simulink model "xpc_dlt_adept_sa_1"  (R2013b)
settings: Solver=ode4  StartTime=0.0  StopTime=4  FixedStep=0.001  RelTol=1e-3
libraries: xpcnilib x6, xpclib x4, simulink x3
(part 1 of 2)
settings Model: BufferReuse=off  Creator=lucius  LastModifiedBy=lucius
settings OptimizationCC: BlockReduction=off  OptimizeBlockIOStorage=off  BufferReuse=off  ExpressionFolding=off  LocalBlockOutputs=off
settings HardwareCC: ProdIntDivRoundTo=Zero  ProdEndianess=LittleEndian  ProdHWDeviceType=Generic->32-bit x86 compatible
settings RTWCC: SystemTargetFile=xpctarget.tlc  TemplateMakefile=xpc_default_tmf  Description=xPC Target  ProcessScript=xpctarget_make_rtw_hook  RTWCompilerOptimization=On
settings xpcTargetCC: TargetFcnLib=ansi_tfl_table_tmw.mat  CodeReplacementLibrary=XPC_BLAS  ParMdlRefBuildCompliant=on  ConcurrentExecutionCompliant=on  CombineSignalStateStructs=off  MATLABClassNameForMDSCustomization=xpcAperiodicCustomization  GRTInterface=on  GenerateAllocFcn=off  xPCTaskExecutionProfile=off  xPCRL32EventNumber=5000  xPCLoadParamSetFile=off  xPCConcurrentTasks=off  xPCEnableSFAnimation=off

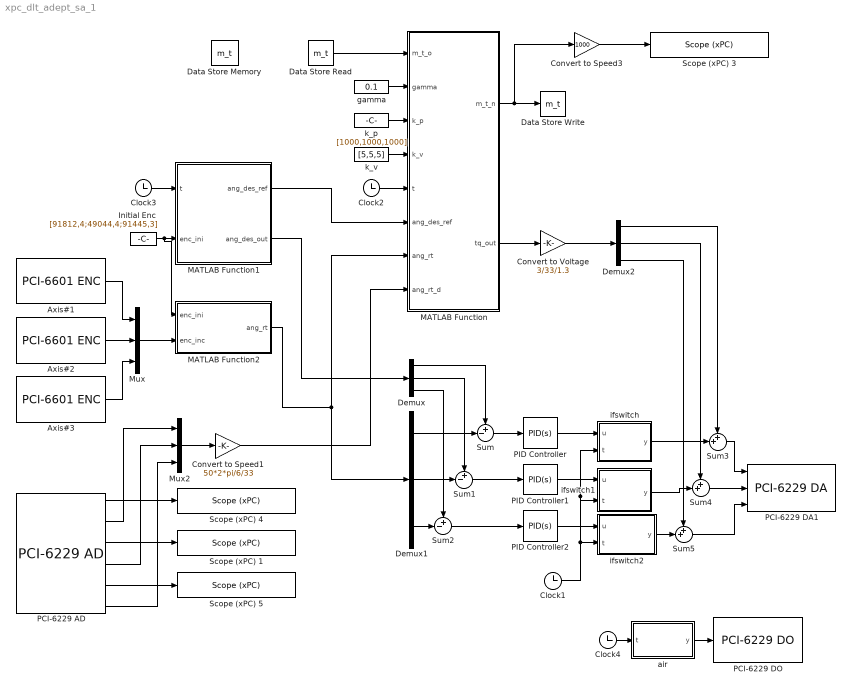
== system xpc_dlt_adept_sa_1 ==
  Axis#1 : xpcnilib/Incremental Encoder/PCI-6601 ENC  channel=1  countMode=Quadrature Mode X4  initCount=0  reload=off  indexPhase=A low B low  filter=None  sampleTime=0.001  slot=-1
  Axis#2 : xpcnilib/Incremental Encoder/PCI-6601 ENC  channel=2  countMode=Quadrature Mode X4  initCount=0  reload=off  indexPhase=A low B low  filter=None  sampleTime=0.001  slot=-1
  Axis#3 : xpcnilib/Incremental Encoder/PCI-6601 ENC  channel=3  countMode=Quadrature Mode X4  initCount=0  reload=off  indexPhase=A low B low  filter=None  sampleTime=0.001  slot=-1
  Clock{1..4} (4 alike) : Clock
  Convert to Speed1 : Gain  Gain=50*2*pi/6/33
  Convert to Speed3 : Gain  Gain=1000
  Convert to Voltage : Gain  Gain=3/33/1.3
  Data Store Memory : DataStoreMemory  DataStoreName=m_t  ReadBeforeWriteMsg=warning  WriteAfterWriteMsg=warning  WriteAfterReadMsg=warning
  Data Store Read : DataStoreRead  DataStoreName=m_t
  Data Store Write : DataStoreWrite  DataStoreName=m_t
  Demux : Demux  Outputs=3
  Demux1 : Demux  Outputs=3
  Demux2 : Demux  Outputs=3
  Initial Enc : Constant  Value=[91812,4;49044,4;91445,3]
  MATLAB Function : MATLAB Function  TreatAsAtomicUnit=on
  MATLAB Function1 : MATLAB Function  TreatAsAtomicUnit=on
  MATLAB Function2 : MATLAB Function  TreatAsAtomicUnit=on
  Mux : Mux  Inputs=3
  Mux2 : Mux  Inputs=3
  PCI-6229 AD : xpcnilib/A//D/M Series/PCI-6229 AD  channel=[1,2,3,4,17,18]  range=[10]  coupling=[0]  scantime=5e-6  sampletime=0.001  slot=-1
  PCI-6229 DA1 : xpcnilib/D//A/M Series/PCI-6229 DA  channel=[1,2,3]  reset=[1,1,1]  initValue=[0,0,0]  sampletime=-1  slot=-1
  PCI-6229 DO : xpcnilib/Digital Output/M Series/PCI-6229 DO  channel=[1]  reset=[1]  initValue=[0]  sampletime=0.001  slot=-1
  PID Controller : simulink/Continuous/PID Controller  Controller=PID  TimeDomain=Continuous-time  SampleTime=1  IntegratorMethod=Forward Euler  FilterMethod=Forward Euler  Form=Parallel  P=50  I=60  D=2  N=100  InitialConditionSource=internal  InitialConditionForIntegrator=0  InitialConditionForFilter=0  ExternalReset=none  LimitOutput=off  UpperSaturationLimit=inf  LowerSaturationLimit=-inf  LinearizeAsGain=on  AntiWindupMode=none  Kb=1  TrackingMode=off  Kt=1  PParamMin=[]  PParamMax=[]  IParamMin=[]  IParamMax=[]  DParamMin=[]  DParamMax=[]  NParamMin=[]  NParamMax=[]  KbParamMin=[]  KbParamMax=[]  KtParamMin=[]  KtParamMax=[]  POutMin=[]  POutMax=[]  IOutMin=[]  IOutMax=[]  DOutMin=[]  DOutMax=[]  NOutMin=[]  NOutMax=[]  KbOutMin=[]  KbOutMax=[]  KtOutMin=[]  KtOutMax=[]  IntegratorOutMin=[]  IntegratorOutMax=[]  FilterOutMin=[]  FilterOutMax=[]  SumOutMin=[]  SumOutMax=[]  SumI1OutMin=[]  SumI1OutMax=[]  SumI2OutMin=[]  SumI2OutMax=[]  SumI3OutMin=[]  SumI3OutMax=[]  SumDOutMin=[]  SumDOutMax=[]  SaturationOutMin=[]  SaturationOutMax=[]  IntegratorContinuousStateAttributes=''  IntegratorStateMustResolveToSignalObject=off  IntegratorRTWStateStorageClass=Auto  FilterContinuousStateAttributes=''  FilterStateMustResolveToSignalObject=off  FilterRTWStateStorageClass=Auto
  PID Controller1 : simulink/Continuous/PID Controller  Controller=PID  TimeDomain=Continuous-time  SampleTime=1  IntegratorMethod=Forward Euler  FilterMethod=Forward Euler  Form=Parallel  P=50  I=60  D=2  N=100  InitialConditionSource=internal  InitialConditionForIntegrator=0  InitialConditionForFilter=0  ExternalReset=none  LimitOutput=off  UpperSaturationLimit=inf  LowerSaturationLimit=-inf  LinearizeAsGain=on  AntiWindupMode=none  Kb=1  TrackingMode=off  Kt=1  PParamMin=[]  PParamMax=[]  IParamMin=[]  IParamMax=[]  DParamMin=[]  DParamMax=[]  NParamMin=[]  NParamMax=[]  KbParamMin=[]  KbParamMax=[]  KtParamMin=[]  KtParamMax=[]  POutMin=[]  POutMax=[]  IOutMin=[]  IOutMax=[]  DOutMin=[]  DOutMax=[]  NOutMin=[]  NOutMax=[]  KbOutMin=[]  KbOutMax=[]  KtOutMin=[]  KtOutMax=[]  IntegratorOutMin=[]  IntegratorOutMax=[]  FilterOutMin=[]  FilterOutMax=[]  SumOutMin=[]  SumOutMax=[]  SumI1OutMin=[]  SumI1OutMax=[]  SumI2OutMin=[]  SumI2OutMax=[]  SumI3OutMin=[]  SumI3OutMax=[]  SumDOutMin=[]  SumDOutMax=[]  SaturationOutMin=[]  SaturationOutMax=[]  IntegratorContinuousStateAttributes=''  IntegratorStateMustResolveToSignalObject=off  IntegratorRTWStateStorageClass=Auto  FilterContinuousStateAttributes=''  FilterStateMustResolveToSignalObject=off  FilterRTWStateStorageClass=Auto
  PID Controller2 : simulink/Continuous/PID Controller  Controller=PID  TimeDomain=Continuous-time  SampleTime=1  IntegratorMethod=Forward Euler  FilterMethod=Forward Euler  Form=Parallel  P=50  I=60  D=2  N=100  InitialConditionSource=internal  InitialConditionForIntegrator=0  InitialConditionForFilter=0  ExternalReset=none  LimitOutput=off  UpperSaturationLimit=inf  LowerSaturationLimit=-inf  LinearizeAsGain=on  AntiWindupMode=none  Kb=1  TrackingMode=off  Kt=1  PParamMin=[]  PParamMax=[]  IParamMin=[]  IParamMax=[]  DParamMin=[]  DParamMax=[]  NParamMin=[]  NParamMax=[]  KbParamMin=[]  KbParamMax=[]  KtParamMin=[]  KtParamMax=[]  POutMin=[]  POutMax=[]  IOutMin=[]  IOutMax=[]  DOutMin=[]  DOutMax=[]  NOutMin=[]  NOutMax=[]  KbOutMin=[]  KbOutMax=[]  KtOutMin=[]  KtOutMax=[]  IntegratorOutMin=[]  IntegratorOutMax=[]  FilterOutMin=[]  FilterOutMax=[]  SumOutMin=[]  SumOutMax=[]  SumI1OutMin=[]  SumI1OutMax=[]  SumI2OutMin=[]  SumI2OutMax=[]  SumI3OutMin=[]  SumI3OutMax=[]  SumDOutMin=[]  SumDOutMax=[]  SaturationOutMin=[]  SaturationOutMax=[]  IntegratorContinuousStateAttributes=''  IntegratorStateMustResolveToSignalObject=off  IntegratorRTWStateStorageClass=Auto  FilterContinuousStateAttributes=''  FilterStateMustResolveToSignalObject=off  FilterRTWStateStorageClass=Auto
  Scope (xPC) 1 : xpclib/Misc./Scope (xPC)   scopeno=5  scopetype=File  autostart=on  viewmode=Graphical redraw  formatstr='%15.6f'  grid=on  ylimits=[0,0]  nosamples=4000  noprepostsamples=0  interleave=1  triggermode=FreeRun  triggersignal=1  trigsignalfromport=off  triggerlevel=0.0  triggerslope=Either  triggerscope=1  triggersample=0  filename=a2t23s12.dat  mode=Lazy  writesize=512  autorestart=off  dynamicfilemode=off  maxwritefilesize=512*1024^2
  Scope (xPC) 3 : xpclib/Misc./Scope (xPC)   scopeno=4  scopetype=File  autostart=on  viewmode=Graphical redraw  formatstr='%15.6f'  grid=on  ylimits=[500,1000]  nosamples=4000  noprepostsamples=0  interleave=1  triggermode=FreeRun  triggersignal=1  trigsignalfromport=off  triggerlevel=0.0  triggerslope=Either  triggerscope=1  triggersample=0  filename=p23s12.dat  mode=Lazy  writesize=512  autorestart=off  dynamicfilemode=off  maxwritefilesize=512*1024^2
  Scope (xPC) 4 : xpclib/Misc./Scope (xPC)   scopeno=1  scopetype=File  autostart=on  viewmode=Graphical redraw  formatstr='%15.6f'  grid=on  ylimits=[0,0]  nosamples=4000  noprepostsamples=0  interleave=1  triggermode=FreeRun  triggersignal=1  trigsignalfromport=off  triggerlevel=0.0  triggerslope=Either  triggerscope=1  triggersample=0  filename=a1t23s12.dat  mode=Lazy  writesize=512  autorestart=off  dynamicfilemode=off  maxwritefilesize=512*1024^2
  Scope (xPC) 5 : xpclib/Misc./Scope (xPC)   scopeno=3  scopetype=File  autostart=on  viewmode=Graphical redraw  formatstr='%15.6f'  grid=on  ylimits=[0,0]  nosamples=4000  noprepostsamples=0  interleave=1  triggermode=FreeRun  triggersignal=1  trigsignalfromport=off  triggerlevel=0.0  triggerslope=Either  triggerscope=1  triggersample=0  filename=a3t23s12.dat  mode=Lazy  writesize=512  autorestart=off  dynamicfilemode=off  maxwritefilesize=512*1024^2
  Sum : Sum  Inputs=+-|
  Sum1 : Sum  Inputs=+-|
  Sum2 : Sum  Inputs=+-|
  Sum3 : Sum  Inputs=++|
  Sum4 : Sum  Inputs=++|
  Sum5 : Sum  Inputs=++|
  air : MATLAB Function  TreatAsAtomicUnit=on
  gamma : Constant  Value=0.1
  ifswitch : MATLAB Function  TreatAsAtomicUnit=on
  ifswitch1 : MATLAB Function  TreatAsAtomicUnit=on
  ifswitch2 : MATLAB Function  TreatAsAtomicUnit=on
  k_p : Constant  Value=[1000,1000,1000]
  k_v : Constant  Value=[5,5,5]
  wires:
  Axis#1/1 -> Mux/1
  Axis#2/1 -> Mux/2
  Axis#3/1 -> Mux/3
  Mux/1 -> MATLAB Function2/2(enc_inc)
  Initial Enc/1 -> MATLAB Function2/1(enc_ini), MATLAB Function1/2(enc_ini)
  Clock3/1 -> MATLAB Function1/1(t)
  MATLAB Function1/1(ang_des_ref) -> MATLAB Function/6(ang_des_ref)
  MATLAB Function/2(tq_out) -> Convert to Voltage/1
  Convert to Voltage/1 -> Demux2/1
  k_v/1 -> MATLAB Function/4(k_v)
  k_p/1 -> MATLAB Function/3(k_p)
  Demux/1 -> Sum/1
  Demux/3 -> Sum2/1
  Demux/2 -> Sum1/1
  Sum/1 -> PID Controller/1
  Sum1/1 -> PID Controller1/1
  Sum2/1 -> PID Controller2/1
  Demux1/1 -> Sum/2
  Demux1/2 -> Sum1/2
  Demux1/3 -> Sum2/2
  Demux2/1 -> Sum3/1
  Demux2/3 -> Sum5/1
  Demux2/2 -> Sum4/1
  Sum3/1 -> PCI-6229 DA1/1
  Sum4/1 -> PCI-6229 DA1/2
  Sum5/1 -> PCI-6229 DA1/3
  PID Controller1/1 -> ifswitch1/1(u)
  PID Controller/1 -> ifswitch/1(u)
  PID Controller2/1 -> ifswitch2/1(u)
  Clock1/1 -> ifswitch/2(t), ifswitch1/2(t), ifswitch2/2(t)
  ifswitch/1(y) -> Sum3/2
  ifswitch1/1(y) -> Sum4/2
  ifswitch2/1(y) -> Sum5/2
  MATLAB Function1/2(ang_des_out) -> Demux/1
  MATLAB Function2/1(ang_rt) -> MATLAB Function/7(ang_rt), Demux1/1
  Clock2/1 -> MATLAB Function/5(t)
  air/1(y) -> PCI-6229 DO/1
  Clock4/1 -> air/1(t)
  gamma/1 -> MATLAB Function/2(gamma)
  Mux2/1 -> Convert to Speed1/1
  PCI-6229 AD/3 -> Scope (xPC) 1/1
  PCI-6229 AD/6 -> Mux2/3
  PCI-6229 AD/4 -> Mux2/2
  PCI-6229 AD/2 -> Mux2/1
  Convert to Speed1/1 -> MATLAB Function/8(ang_rt_d)
  MATLAB Function/1(m_t_n) -> Convert to Speed3/1, Data Store Write/1
  Data Store Read/1 -> MATLAB Function/1(m_t_o)
  Convert to Speed3/1 -> Scope (xPC) 3/1
  PCI-6229 AD/1 -> Scope (xPC) 4/1
  PCI-6229 AD/5 -> Scope (xPC) 5/1

== matlab function xpc_dlt_adept_sa_1/ifswitch1 ==
  data: u input; y output; t input
function y = ifswitch(u,t)
T=2;
if t<T
y = u;
else y=0;
end

== matlab function xpc_dlt_adept_sa_1/ifswitch ==
  data: u input; y output; t input
function y = ifswitch(u,t)
T=2;
if t<T
y = u;
else y=0;
end

== matlab function xpc_dlt_adept_sa_1/MATLAB Function2 ==
  data: enc_ini input; ang_rt output; enc_inc input
function ang_rt = inc2jo(enc_ini,enc_inc)
%***********************REFERENCE****************************************
%LIMIT&ABSOLUTE NUMBER
%Axis#      Limit   Absolute Position
%1          -45     14circles   +1784
%           100     0circles    +98713

%2          -45     13circles   +120485
%           100     0circles    +87782

%3          -45     13circles   +77696
%           100     0circles    +44275

%************************COMPUTATION**************************************
enc_rt=[0,0,0];
enc_rt(1)=enc_ini(1,2)*131072+enc_ini(1,1)+enc_inc(1)*131072/10000;%real time
enc_rt(2)=enc_ini(2,2)*131072+enc_ini(2,1)+enc_inc(2)*131072/10000;%encoder
enc_rt(3)=enc_ini(3,2)*131072+enc_ini(3,1)+enc_inc(3)*131072/10000;%value
ang_rt=[0;0;0];
%Axis#1
ang_rt(1)=(enc_rt(1)-98713)*pi*29/36/(14*131072+1784-98713)-5*pi/9;
%Axis#2
ang_rt(2)=(enc_rt(2)-87782)*pi*29/36/(13*131072+120485-87782)-5*pi/9;
%Axis#3
ang_rt(3)=(enc_rt(3)-44275)*pi*29/36/(13*131072+77696-44275)-5*pi/9;

== matlab function xpc_dlt_adept_sa_1/MATLAB Function ==
  data: m_t_o input; m_t_n output; gamma input; k_p input; k_v input; t input; tq_out output; ang_des_ref input; ang_rt input; ang_rt_d input
function [m_t_n,tq_out] = dcal(m_t_o,gamma,k_p,k_v,t,ang_des_ref,ang_rt,ang_rt_d)
T=2;
if t<T
    tq_out=[0;0;0];
    m_t_n=0;
else
    % PARAMETER
    % /**********************************************************************/
    %GEOMETRY
    L_A=270/1000;                %length of the drive link
    C_R=33;                      %reductor coefficient
    
    %INERTIA
    G=9.8;                  %gravity acceleration
    I_R=0.22;                   %inertia of the reductor
    I_M=(I_R+0.26)*10^(-4)*C_R^2;  %inertia of the motor and reductor(convert to output axis)
    M_A=0.8806;             %mass of the drive link
    M_E=0.21;%0.064;              %mass of elbow
    M_F=0.490;                %mass of the passive link
    %M_T=0.710;                  %mass of the travelling plate
    F_V=diag([3.25,1.16,1.32]);                 %viscous friction coefficients
    F_C=diag([2.13,1.74,3.17]);                 %Coulomb friction
    C_A=diag([0.08,0.19,0.1]);                 %acceleration compensation
    %ERROR
    % /***********************************************************************/
    ang_rt_local=-[ang_rt(1);ang_rt(3);ang_rt(2)];
    ang_rt_d_local=-[ang_rt_d(1);ang_rt_d(3);ang_rt_d(2)];
    err_ang=[ang_des_ref(1);ang_des_ref(2);ang_des_ref(3)]-ang_rt_local;
    err_ang_d=[ang_des_ref(4);ang_des_ref(5);ang_des_ref(6)]-ang_rt_d_local;
    err_filt=[k_p(1)*err_ang(1);k_p(2)*err_ang(2);k_p(3)*err_ang(3)]...
        +[k_v(1)*err_ang_d(1);k_v(2)*err_ang_d(2);k_v(3)*err_ang_d(3)];
    %UPDATER
    % /***********************************************************************/
    jc=dltjc([ang_des_ref(1);ang_des_ref(2);ang_des_ref(3)]);
    stp=0.001;%simulate step
    m_t_n=gamma*[ang_des_ref(10),ang_des_ref(11),ang_des_ref(12)-G]*jc*err_filt*stp+m_t_o;
    %ADAPTIVE CONTROLLER
    % /***********************************************************************/
    i_aci=I_M+L_A^2*(M_A/3+M_E+M_F*2/3);
    i_ac=diag([i_aci,i_aci,i_aci])+C_A;
    g_ac=(M_A/2+M_E+M_F/2)*L_A*G*cos([ang_des_ref(1);ang_des_ref(2);ang_des_ref(3)]);
    torq=i_ac*[ang_des_ref(7);ang_des_ref(8);ang_des_ref(9)]-g_ac...
        +M_F*jc'*[ang_des_ref(10);ang_des_ref(11);ang_des_ref(12)-1.5*G]...
        +F_V*[ang_des_ref(4);ang_des_ref(5);ang_des_ref(6)]+F_C*sign([ang_des_ref(4);ang_des_ref(5);ang_des_ref(6)])...
        +jc'*[ang_des_ref(10);ang_des_ref(11);ang_des_ref(12)-G]*m_t_n...
        +err_filt;
    tq_out=-[torq(1);torq(3);torq(2)];%convert to the real torq comand
end

== matlab function xpc_dlt_adept_sa_1/ifswitch2 ==
  data: u input; y output; t input
function y = ifswitch(u,t)
T=2;
if t<T
y = u;
else y=0;
end

== matlab function xpc_dlt_adept_sa_1/air ==
  data: y output; t input
function y = airon(t)
if t>3
   y = 1;
else
   y=0;
end
